simulink model "debug_FTMeas_shoes"  (Simulink 9.0)
settings: Solver=FixedStepDiscrete  StartTime=0.0  StopTime=inf  FixedStep=0.01  RelTol=1e-3  EnableMultiTasking=on
InitFcn:
  | ROBOT_DOF=23;
libraries: WBToolboxLibrary x9
settings Model: SuppressorTable=22 serialization::archive 11 0 6 0 0 0 1 0  Creator=DanielePucci  LastModifiedBy=gnava
settings DataIOCC: LimitDataPoints=on  SaveFormat=Dataset
settings DebuggingCC: UnderspecifiedInitializationDetection=Simplified  MergeDetectMultiDrivingBlocksExec=error  AllowSymbolicDim=off
settings HardwareCC: ProdBitPerPointer=64  ProdBitPerSizeT=64  ProdBitPerPtrDiffT=64  ProdLargestAtomicFloat=Float  ProdIntDivRoundTo=Zero  ProdEndianess=LittleEndian  ProdWordSize=64  ProdHWDeviceType=Intel->x86-64 (Windows64)

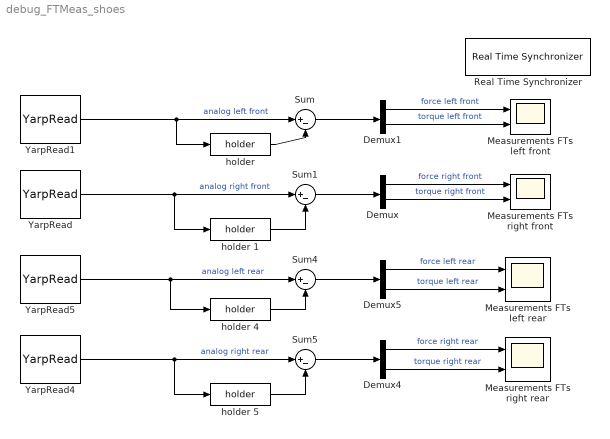
== system debug_FTMeas_shoes ==
  Demux{,1,4..5} (4 alike) : Demux  Outputs=2
  Measurements FTs left front : Scope  NumInputPorts=2
  Measurements FTs left rear : Scope  NumInputPorts=2
  Measurements FTs right front : Scope  NumInputPorts=2
  Measurements FTs right rear : Scope  NumInputPorts=2
  Real Time Synchronizer : WBToolboxLibrary/Utilities/Real Time Synchronizer  period=0.01
      settings: SourceProductName=WholeBodyToolbox
  Sum{,1,4..5} (4 alike) : Sum  Inputs=|+-
  YarpRead : WBToolboxLibrary/Utilities/YarpRead  portName='ft/ftShoe_Right_Front/analog:o'  signalSize=6  timeout=0.5  blocking=off  timestamp=off  autoconnect=on  errorOnConnection=off
      settings: SourceProductName=WholeBodyToolbox
  YarpRead1 : WBToolboxLibrary/Utilities/YarpRead  portName='ft/ftShoe_Left_Front/analog:o'  signalSize=6  timeout=0.5  blocking=off  timestamp=off  autoconnect=on  errorOnConnection=off
      settings: SourceProductName=WholeBodyToolbox
  YarpRead4 : WBToolboxLibrary/Utilities/YarpRead  portName='ft/ftShoe_Right_Rear/analog:o'  signalSize=6  timeout=0.5  blocking=off  timestamp=off  autoconnect=on  errorOnConnection=off
      settings: SourceProductName=WholeBodyToolbox
  YarpRead5 : WBToolboxLibrary/Utilities/YarpRead  portName='ft/ftShoe_Left_Rear/analog:o'  signalSize=6  timeout=0.5  blocking=off  timestamp=off  autoconnect=on  errorOnConnection=off
      settings: SourceProductName=WholeBodyToolbox
  holder {,1,4..5} (4 alike) : WBToolboxLibrary/Utilities/holder 
      settings: SourceProductName=WholeBodyToolbox
  wires:
  YarpRead/1 -> holder 1/1, Sum1/1  "analog right front"
  Demux/1 -> Measurements FTs right front/1  "force right front"
  Demux/2 -> Measurements FTs right front/2  "torque right front"
  YarpRead1/1 -> Sum/1, "holder "/1  "analog left front"
  Demux1/1 -> Measurements FTs left front/1  "force left front"
  Demux1/2 -> Measurements FTs left front/2  "torque left front"
  "holder "/1 -> Sum/2
  Sum/1 -> Demux1/1
  holder 1/1 -> Sum1/2
  Sum1/1 -> Demux/1
  YarpRead4/1 -> holder 5/1, Sum5/1  "analog right rear"
  Demux4/1 -> Measurements FTs right rear/1  "force right rear"
  Demux4/2 -> Measurements FTs right rear/2  "torque right rear"
  YarpRead5/1 -> Sum4/1, holder 4/1  "analog left rear"
  Demux5/2 -> Measurements FTs left rear/2  "torque left rear"
  holder 4/1 -> Sum4/2
  Sum4/1 -> Demux5/1
  holder 5/1 -> Sum5/2
  Sum5/1 -> Demux4/1
  Demux5/1 -> Measurements FTs left rear/1  "force left rear"
